simulink model "V2_3"  (R2023b)
settings: Solver=FixedStepAuto  StartTime=0.0  StopTime=inf  RelTol=1e-3
libraries: robotlib x14
settings Model: PacingRate=100  Creator=Renzhaofu  LastModifiedBy=Renzhaofu
settings OptimizationCC: EnhancedBackFolding=on  PassReuseOutputArgsAs=Individual arguments  ZeroExternalMemoryAtStartup=off  ZeroInternalMemoryAtStartup=off  MaxStackSize=64  OptimizeBlockOrder=speed  DifferentSizesBufferReuse=on  OptimizationCustomize=off  EfficientTunableParamExpr=on
settings DebuggingCC: ParameterTunabilityLossMsg=error
settings HardwareCC: ProdBitPerPointer=32  ProdBitPerSizeT=32  ProdBitPerPtrDiffT=32  ProdLargestAtomicFloat=None  ProdIntDivRoundTo=Undefined  ProdEndianess=Unspecified  ProdWordSize=32  ProdHWDeviceType=Generic->Unspecified (assume 32-bit Generic)
settings SFSimCC: MATLABDynamicMemAlloc=off
settings RTWCC: Description=Embedded Coder  SystemTargetFile=ert.tlc  HardwareBoard=Robot Operating System (ROS)  TLCOptions="-aInlineSetEventsForThisBaseRateFcn=TLC_FALSE -aSuppressMultiTaskScheduler=TLC_FALSE  -aRateBasedStepFcn=0"  TemplateMakefile=ert_default_tmf  Toolchain=Catkin  TargetLang=C++
settings CodeAppCC: ForceParamTrailComments=on  IgnoreCustomStorageClasses=off  OperatorAnnotations=on  SimulinkDataObjDesc=on  SFDataObjDesc=on  InsertBlockDesc=on

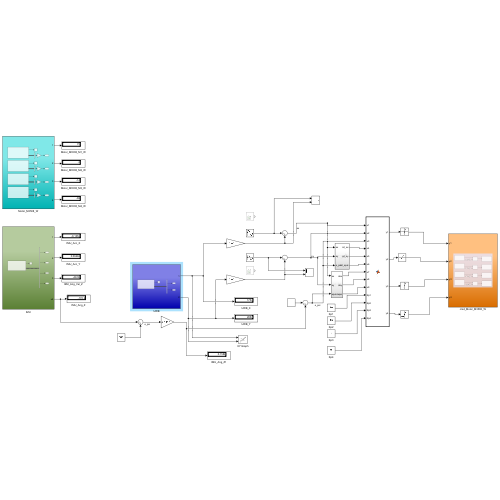
[thumbnail: Simulink's stored preview of the top-level diagram]
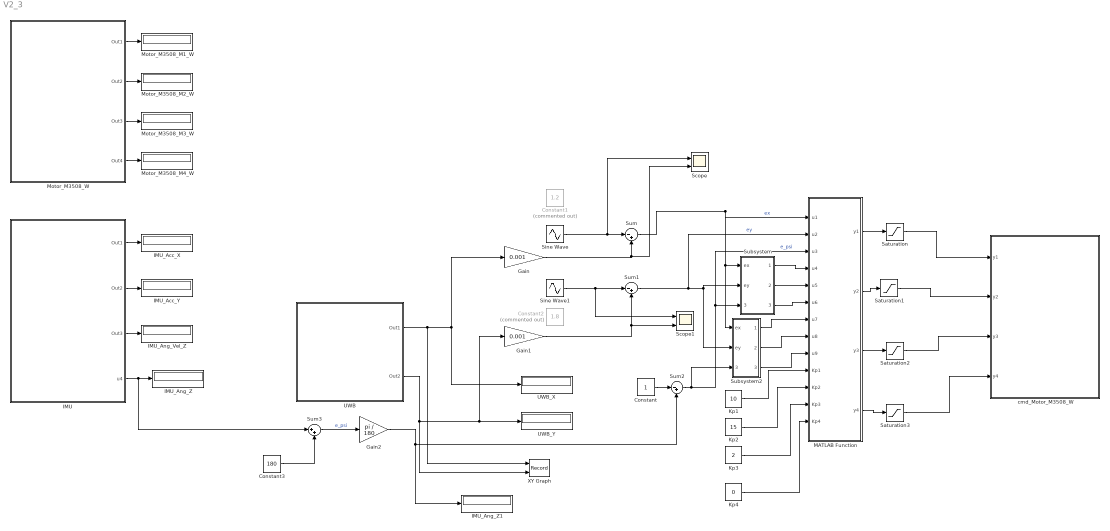
== system V2_3 ==
  Constant : Constant
  Constant1 : Constant  Commented=on  Value=1.2
  Constant2 : Constant  Commented=on  Value=1.8
  Constant3 : Constant  Value=180
  Gain : Gain  Gain=0.001
  Gain1 : Gain  Gain=0.001
  Gain2 : Gain  Gain=pi / 180
  IMU : Subsystem
  IMU_Acc_X : Display
  IMU_Acc_Y : Display
  IMU_Ang_Vel_Z : Display
  IMU_Ang_Z : Display
  IMU_Ang_Z1 : Display
  Kp1 : Constant  Value=10
  Kp2 : Constant  Value=15
  Kp3 : Constant  Value=2
  Kp4 : Constant  Value=0
  MATLAB Function : MATLAB Function  TreatAsAtomicUnit=on
  Motor_M3508_M1_W : Display
  Motor_M3508_M2_W : Display
  Motor_M3508_M3_W : Display
  Motor_M3508_M4_W : Display
  Motor_M3508_W : Subsystem
  Saturation{,1..3} (4 alike) : Saturate  UpperLimit=75  LowerLimit=-75  OutDataTypeStr=single
  Scope : Scope  NumInputPorts=2
  Scope1 : Scope  NumInputPorts=2
  Sine Wave : Sin  Amplitude=0.1  Bias=1.2  Frequency=0.1  SampleTime=0
  Sine Wave1 : Sin  Amplitude=0.1  Bias=1.2  Frequency=0.1  Phase=pi/2  SampleTime=0
  Subsystem : Subsystem
  Subsystem2 : Subsystem
  Sum : Sum  Inputs=|-+
  Sum1 : Sum  Inputs=|-+
  Sum2 : Sum  Inputs=|-+
  Sum3 : Sum  Inputs=|++
  UWB : Subsystem
  "UWB_X " : Display
  UWB_Y : Display
  XY Graph : Record  FileSettingsInternal="{\"entries\":[{\"content\":{\"excelSettings\":{\"content\":{},\"type\":\"Streamout.ExcelSettings\"}},\"type\":\"Streamout.FileSettingStorage\",\"uuid\":\"\"}],\"packageUris\":[\"http:\\/\\/schema.mathworks.com\\/mf0\\/streamout_blocks\\/R2020a\"],\"version\":\"1.0\"}"  Layout=[1 1]  SignalsInternal="{\"entries\":[{\"content\":{\"signals\":[{\"content\":{\"blockPath\":[],\"dimensions\":[1],\"domain\":\"\",\"lineColor\":\"#a2142f\",\"port\":1,\"sid\":[\"\"],\"signalID\":388,\"signalName\":\"UWB:1\"},\"type\":\"RecordBlkView.Signal\",\"uuid\":\"\"},{\"content\":{\"blockPath\":[],\"dimensions\":[1],\"domain\":\"\",\"lineColor\":\"#139fff\",\"port\":2,\"sid\":[\"\"],\"signalID\":392,\"signalName\":\"UWB:2\"},\"type\":\"RecordBlkView.Signal\",\"uuid\":\"\"}]},\"type\":\"RecordBlkView.InputSignals\",\"uuid\":\"\"}],\"packageUris\":[\"http:\\/\\/schema.mathworks.com\\/mf0\\/streamout_blocks\\/R2020a\"],\"version\":\"1.0\"}"  VisualizationBindings="{\"xyplotplugin\":{\"info\":[{\"series\":[],\"subplotID\":1}]}}"  CompatibilityTag=XY
  cmd_Motor_M3508_W : Subsystem
  wires:
  IMU/1(Out1) -> IMU_Acc_X/1
  IMU/2(Out2) -> IMU_Acc_Y/1
  IMU/3(Out3) -> IMU_Ang_Vel_Z/1
  IMU/4(u4) -> Sum3/1, IMU_Ang_Z/1
  UWB/1(Out1) -> XY Graph/1, Gain/1, "UWB_X "/1
  UWB/2(Out2) -> XY Graph/2, Gain1/1, UWB_Y/1
  Sum/1 -> MATLAB Function/1(u1), Subsystem2/1(ex), Subsystem/1(ex)  "ex"
  Sum1/1 -> MATLAB Function/2(u2), Subsystem2/2(ey), Subsystem/2(ey)  "ey"
  Constant/1 -> Sum2/1
  Sum2/1 -> Subsystem2/3(epsi), MATLAB Function/3(u3), Subsystem/3(e_psi)  "e_psi"
  MATLAB Function/1(y1) -> Saturation/1
  MATLAB Function/3(y3) -> Saturation2/1
  Motor_M3508_W/3(Out3) -> Motor_M3508_M3_W/1
  Motor_M3508_W/1(Out1) -> Motor_M3508_M1_W/1
  Motor_M3508_W/2(Out2) -> Motor_M3508_M2_W/1
  Motor_M3508_W/4(Out4) -> Motor_M3508_M4_W/1
  Saturation/1 -> cmd_Motor_M3508_W/1(y1)
  Saturation3/1 -> cmd_Motor_M3508_W/4(y4)
  Saturation2/1 -> cmd_Motor_M3508_W/3(y3)
  Saturation1/1 -> cmd_Motor_M3508_W/2(y2)
  MATLAB Function/2(y2) -> Saturation1/1
  MATLAB Function/4(y4) -> Saturation3/1
  Gain/1 -> Scope/2, Sum/2
  Gain1/1 -> Scope1/2, Sum1/2
  Constant3/1 -> Sum3/2
  Sum3/1 -> Gain2/1  "e_psi"
  Gain2/1 -> IMU_Ang_Z1/1, Sum2/2
  Subsystem/1(int_ex) -> MATLAB Function/4(u4)
  Subsystem/2(int_ey) -> MATLAB Function/5(u5)
  Subsystem/3(int_epsi) -> MATLAB Function/6(u6)
  Sine Wave/1 -> Scope/1, Sum/1
  Sine Wave1/1 -> Scope1/1, Sum1/1
  Subsystem2/1(dex) -> MATLAB Function/7(u7)
  Subsystem2/2(dey) -> MATLAB Function/8(u8)
  Subsystem2/3(depsi) -> MATLAB Function/9(u9)
  Kp1/1 -> MATLAB Function/10(Kp1)
  Kp2/1 -> MATLAB Function/11(Kp2)
  Kp3/1 -> MATLAB Function/12(Kp3)
  Kp4/1 -> MATLAB Function/13(Kp4)

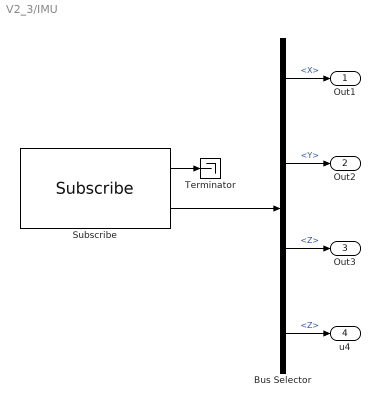
== system V2_3/IMU ==
  Bus Selector : BusSelector  OutputSignals=LinearAcceleration.X,LinearAcceleration.Y,AngularVelocity.Z,Orientation.Z
  Subscribe : robotlib/Subscribe  topicSource=Select from ROS network  topic=/IMU_Topic  messageType=sensor_msgs/Imu  SampleTime=0.001  legacyBusStruct=off  messageQueueLength=1
  Terminator : Terminator
  Out1 : Outport
  Out2 : Outport  Port=2
  Out3 : Outport  Port=3
  u4 : Outport  Port=4
  wires:
  Bus Selector/3 -> Out3/1  "<Z>"
  Subscribe/2 -> Bus Selector/1
  Subscribe/1 -> Terminator/1
  Bus Selector/4 -> u4/1  "<Z>"
  Bus Selector/2 -> Out2/1  "<Y>"
  Bus Selector/1 -> Out1/1  "<X>"

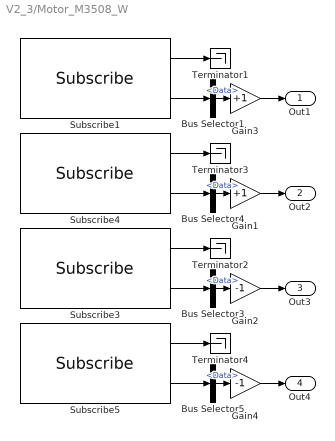
== system V2_3/Motor_M3508_W ==
  Bus Selector{1,3..5} (4 alike) : BusSelector  OutputSignals=Data
  Gain1 : Gain  Gain=+1
  Gain2 : Gain  Gain=-1
  Gain3 : Gain  Gain=+1
  Gain4 : Gain  Gain=-1
  Subscribe1 : robotlib/Subscribe  topicSource=Select from ROS network  topic=/Motor_M3508_M1_W_Topic  messageType=std_msgs/Float32  SampleTime=0.001  legacyBusStruct=off  messageQueueLength=1
  Subscribe3 : robotlib/Subscribe  topicSource=Select from ROS network  topic=/Motor_M3508_M3_W_Topic  messageType=std_msgs/Float32  SampleTime=0.001  legacyBusStruct=off  messageQueueLength=1
  Subscribe4 : robotlib/Subscribe  topicSource=Select from ROS network  topic=/Motor_M3508_M2_W_Topic  messageType=std_msgs/Float32  SampleTime=0.001  legacyBusStruct=off  messageQueueLength=1
  Subscribe5 : robotlib/Subscribe  topicSource=Select from ROS network  topic=/Motor_M3508_M4_W_Topic  messageType=std_msgs/Float32  SampleTime=0.001  legacyBusStruct=off  messageQueueLength=1
  Terminator{1..4} (4 alike) : Terminator
  Out1 : Outport
  Out2 : Outport  Port=2
  Out3 : Outport  Port=3
  Out4 : Outport  Port=4
  wires:
  Subscribe5/2 -> Bus Selector5/1
  Subscribe1/1 -> Terminator1/1
  Subscribe1/2 -> Bus Selector1/1
  Subscribe3/1 -> Terminator2/1
  Subscribe4/1 -> Terminator3/1
  Subscribe4/2 -> Bus Selector4/1
  Subscribe3/2 -> Bus Selector3/1
  Subscribe5/1 -> Terminator4/1
  Gain3/1 -> Out1/1
  Bus Selector1/1 -> Gain3/1  "<Data>"
  Bus Selector5/1 -> Gain4/1  "<Data>"
  Bus Selector3/1 -> Gain2/1  "<Data>"
  Bus Selector4/1 -> Gain1/1  "<Data>"
  Gain1/1 -> Out2/1
  Gain2/1 -> Out3/1
  Gain4/1 -> Out4/1

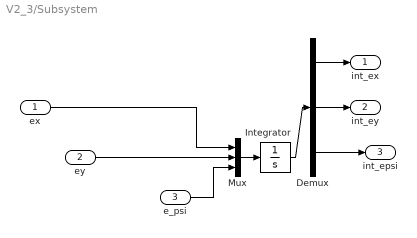
== system V2_3/Subsystem ==
  ex : Inport
  ey : Inport  Port=2
  e_psi : Inport  Port=3
  Demux : Demux  Outputs=3
  Integrator : Integrator
  Mux : Mux  Inputs=3
  int_ex : Outport
  int_ey : Outport  Port=2
  int_epsi : Outport  Port=3
  wires:
  Mux/1 -> Integrator/1
  Demux/3 -> int_epsi/1
  ex/1 -> Mux/1
  e_psi/1 -> Mux/3
  Integrator/1 -> Demux/1
  Demux/2 -> int_ey/1
  ey/1 -> Mux/2
  Demux/1 -> int_ex/1

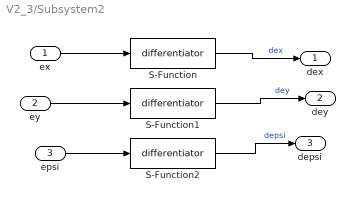
== system V2_3/Subsystem2 ==
  ex : Inport
  ey : Inport  Port=2
  epsi : Inport  Port=3
  S-Function : S-Function  FunctionName=differentiator  SFunctionDeploymentMode=off  EnableBusSupport=off
  S-Function1 : S-Function  FunctionName=differentiator  SFunctionDeploymentMode=off  EnableBusSupport=off
  S-Function2 : S-Function  FunctionName=differentiator  SFunctionDeploymentMode=off  EnableBusSupport=off
  dex : Outport
  dey : Outport  Port=2
  depsi : Outport  Port=3
  wires:
  ey/1 -> S-Function1/1
  S-Function/1 -> dex/1  "dex"
  epsi/1 -> S-Function2/1
  S-Function1/1 -> dey/1  "dey"
  S-Function2/1 -> depsi/1  "depsi"
  ex/1 -> S-Function/1

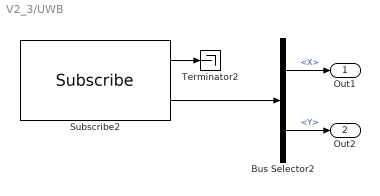
== system V2_3/UWB ==
  Bus Selector2 : BusSelector  OutputSignals=X,Y
  Subscribe2 : robotlib/Subscribe  topicSource=Select from ROS network  topic=/UWB_Topic  messageType=geometry_msgs/Point  SampleTime=0.001  legacyBusStruct=off  messageQueueLength=1
  Terminator2 : Terminator
  Out1 : Outport
  Out2 : Outport  Port=2
  wires:
  Bus Selector2/1 -> Out1/1  "<X>"
  Subscribe2/2 -> Bus Selector2/1
  Subscribe2/1 -> Terminator2/1
  Bus Selector2/2 -> Out2/1  "<Y>"

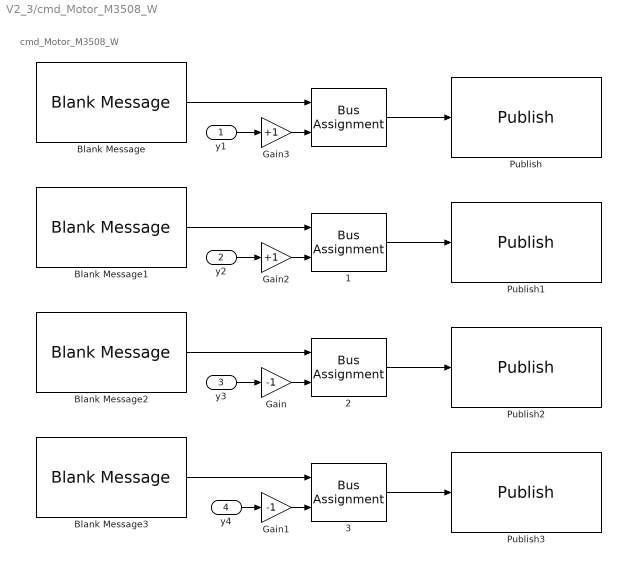
== system V2_3/cmd_Motor_M3508_W ==
  note: cmd_Motor_M3508_W
  y1 : Inport
  y2 : Inport  Port=2
  y3 : Inport  Port=3
  y4 : Inport  Port=4
   {,1..3} (4 alike) : BusAssignment  AssignedSignals=Data
  Blank Message{,1..3} (4 alike) : robotlib/Blank Message  messageClass=Message  entityType=std_msgs/Float32  messageType=std_msgs/Float32  SampleTime=inf  legacyBusStruct=off
  Gain : Gain  Gain=-1
  Gain1 : Gain  Gain=-1
  Gain2 : Gain  Gain=+1
  Gain3 : Gain  Gain=+1
  Publish : robotlib/Publish  topicSource=Select from ROS network  topic=/cmd_Motor_M3508_M1_W  messageType=std_msgs/Float32  legacyBusStruct=off  messageQueueLength=1
  Publish1 : robotlib/Publish  topicSource=Select from ROS network  topic=/cmd_Motor_M3508_M2_W  messageType=std_msgs/Float32  legacyBusStruct=off  messageQueueLength=1
  Publish2 : robotlib/Publish  topicSource=Select from ROS network  topic=/cmd_Motor_M3508_M3_W  messageType=std_msgs/Float32  legacyBusStruct=off  messageQueueLength=1
  Publish3 : robotlib/Publish  topicSource=Select from ROS network  topic=/cmd_Motor_M3508_M4_W  messageType=std_msgs/Float32  legacyBusStruct=off  messageQueueLength=1
  wires:
  Blank Message/1 -> " "/1
  " 3"/1 -> Publish3/1
  " 2"/1 -> Publish2/1
  y1/1 -> Gain3/1
  Gain2/1 -> " 1"/2
  Blank Message3/1 -> " 3"/1
  " "/1 -> Publish/1
  Blank Message2/1 -> " 2"/1
  y3/1 -> Gain/1
  Gain/1 -> " 2"/2
  Gain3/1 -> " "/2
  " 1"/1 -> Publish1/1
  Blank Message1/1 -> " 1"/1
  y2/1 -> Gain2/1
  Gain1/1 -> " 3"/2
  y4/1 -> Gain1/1

== matlab function V2_3/MATLAB Function ==
  data: u1 input; y1 output; u2 input; u3 input; y2 output; y3 output; y4 output; u4 input; u5 input; u6 input; u7 input; u8 input; u9 input; Kp1 input; Kp2 input; Kp3 input; Kp4 input
function [y1, y2, y3, y4] = fcn(u1,u2,u3,u4,u5,u6,u7,u8,u9,Kp1,Kp2,Kp3,Kp4)

%%%%%%%%%%%%%% 注意： u1,u2,u3 分别为地球坐标系下的 x轴的跟踪误差，y轴的跟踪误差，偏航角跟踪误差 %%%%%%%%%%%%%%
a = 0.150;  %%%%%%%%%%%%% a是（一半）车宽长度（单位：MM） %%%%%%%%%%%%%
b = 0.120;  %%%%%%%%%%%%% b是（一半）一侧两麦轮轴间距（单位：MM）%%%%%%%%%%%%%

psi = u3 + pi/4;

ee = [u1;u2;u3];
jifen_ee = [u4;u5;u6];
weifen_ee = [u7;u8;u9];

H=[(2^0.5)*sin(psi), -(2^0.5)*cos(psi), -a-b; (2^0.5)*cos(psi),(2^0.5)*sin(psi),-a-b; (2^0.5)*sin(psi), -(2^0.5)*cos(psi), a+b;(2^0.5)*cos(psi),(2^0.5)*sin(psi),a+b];

%Kp1 = kp1;
%Kp2 = kp2;
%Kp3 = Kp3;
% kp4 = 2;

y = -Kp1 .* H * ee - Kp2 .* H * sign(ee) - Kp3 .* H * jifen_ee - Kp4 .* H * weifen_ee;
% y = -Kp1 .* H * ee - Kp2 .* H * sign(ee) - Kp3 .* H * jifen_ee;

y1 = y(1);
y2 = y(2);
y3 = y(3);
y4 = y(4);
